simulink model "model1"  (R2024a)
settings: Solver=VariableStepAuto  StartTime=0.0  StopTime=simulation_time  RelTol=1e-3
values from neighbouring files (symbols this model uses):
  dq_0 = zeros(n, 1)    [example.m]
  path = @(t) circle_center + u_circle_plane*radius*cos((t/T) * (2*pi)) + v_circle_plane*radius*sin((t/T) * (2*pi))    [example.m]
  path_ddot = @(t) -u_circle_plane*radius*(2*pi/T)*(2*pi/T)*cos((t/T) * (2*pi)) - v_circle_plane*radius*(2*pi/T)*(2*pi/T)*sin((t/T) * (2*pi))    [example.m]
  path_dot = @(t) -u_circle_plane*radius*(2*pi/T)*sin((t/T) * (2*pi)) + v_circle_plane*radius*(2*pi/T)*cos((t/T) * (2*pi))    [example.m]
  q_0 = randn(n, 1)    [example.m]
  robot_model = importrobot("../robot_model/kuka-lwr-4plus/model1.urdf", 'DataFormat', 'column')    [example.m]
undefined symbols (not defined in the file or in its folder): torque_low_bound, torque_up_bound, X, Y, Z
libraries: sm_lib x74, nesl_utility x8, robotmaniplib x4
(part 3 of 5)

== matlab function model1/MATLAB Function4 ==
  data: currJointPos input; M_num output
function M_num = M_num1(currJointPos)
%M_num1
%    M_num = M_num1(Q2,Q3,Q4,Q5,Q6,Q7)

%    This function was generated by the Symbolic Math Toolbox version 24.1.
%    01-Jul-2024 12:17:03

q2 = currJointPos(2);
q3 = currJointPos(3);
q4 = currJointPos(4);
q5 = currJointPos(5);
q6 = currJointPos(6);
q7 = currJointPos(7);

t2 = cos(q2);
t3 = cos(q3);
t4 = cos(q4);
t5 = cos(q5);
t6 = cos(q6);
t7 = cos(q7);
t8 = sin(q2);
t9 = sin(q3);
t10 = sin(q4);
t11 = sin(q5);
t12 = sin(q6);
t13 = sin(q7);
t14 = t3.^2;
t15 = t4.^2;
t16 = t5.^2;
t17 = t6.^2;
t18 = t7.^2;
t19 = t8.^2;
t20 = t9.^2;
t21 = t10.^2;
t22 = t11.^2;
t23 = t12.^2;
t24 = t13.^2;
t25 = t2.*t4;
t26 = t3.*t5;
t27 = t4.*t6;
t28 = t5.*t7;
t29 = t2.*t10;
t30 = t3.*t11;
t31 = t4.*t12;
t32 = t5.*t13;
t33 = t9.*(2.0./5.0);
t34 = t8.*t9.*t11;
t35 = t9.*t10.*t12;
t36 = t10.*t11.*t13;
t37 = t3.*t4.*t8;
t38 = t4.*t5.*t9;
t39 = t5.*t6.*t10;
t40 = t6.*t7.*t11;
t41 = t3.*t8.*t10;
t42 = t5.*t8.*t9;
t43 = t4.*t9.*t11;
t44 = t6.*t9.*t10;
t45 = t5.*t10.*t12;
t46 = t7.*t10.*t11;
t47 = t6.*t11.*t13;
t48 = t3.*t4.*(2.0./5.0);
t49 = t3.*t8.*(2.0./5.0);
t50 = t3.*t10.*(2.0./5.0);
t53 = t3.*(7.0./1.0e+2);
t57 = t4.*t9.*(3.0./5.0e+1);
t58 = t9.*t11.*(-2.0./5.0);
t59 = t9.*t10.*(3.0./5.0e+1);
t60 = t2.*(1.3e+1./1.0e+2);
t61 = t4.*(3.1e+1./2.5e+2);
t69 = t3.*t4.*(7.0./1.25e+2);
t72 = t4.*t9.*(7.0./1.0e+2);
t74 = t8.*t9.*(2.3e+1./5.0e+1);
t75 = t8.*t9.*(7.0./1.0e+2);
t76 = t2.*1.68e-2;
t77 = t4.*1.68e-2;
t78 = t3.*4.2e-3;
t79 = t2.*7.8e-3;
t80 = t6.*1.2e-4;
t92 = t8.*t9.*t10.*(-2.0./5.0);
t95 = t7.*t11.*(3.9e+1./1.0e+2);
t97 = t10.*t11.*(3.9e+1./1.0e+2);
t98 = t11.*t13.*(3.9e+1./1.0e+2);
t99 = t9.*t10.*(3.1e+1./2.5e+2);
t102 = t3.*1.352e-1;
t104 = t3.*t6.*t10.*(-2.0./5.0);
t114 = t9.*t11.*(6.2e+1./6.25e+2);
t115 = t9.*t10.*1.68e-2;
t116 = t8.*t9.*4.2e-3;
t117 = t9.*t10.*4.2e-3;
t118 = t11.*t12.*1.2e-4;
t125 = t4.*t8.*t9.*(7.0./1.25e+2);
t130 = t8.*t9.*1.352e-1;
t132 = t8.*t9.*5.1e-3;
t133 = t9.*t10.*5.1e-3;
t135 = t5.*9.672e-2;
t173 = t10.*t11.*9.672e-2;
t261 = t3.*1.083333333335e-2;
t267 = t8.*t9.*1.083333333335e-2;
t289 = t5.*2.6708333333367e-3;
t291 = t3.*3.14666666667e-2;
t303 = t2.*7.94666666667e-2;
t308 = t10.*t11.*2.6708333333367e-3;
t309 = t8.*t9.*3.14666666667e-2;
t329 = t3.*t8.*t9.*5.065666666667e-1;
t339 = t4.*t9.*t10.*1.603599999999999e-2;
t352 = t6.*t11.*t12.*5.33333333333e-5;
t358 = t4.*7.50255000000367e-2;
t377 = t9.*t10.*7.50255000000367e-2;
t402 = t5.*t10.*t11.*7.12080000000333e-2;
t51 = t5.*t33;
t52 = t11.*t33;
t54 = t25.*(3.0./5.0e+1);
t55 = -t50;
t56 = t29.*(3.0./5.0e+1);
t62 = -t37;
t63 = -t39;
t65 = -t43;
t68 = -t47;
t70 = t8.*t10.*t33;
t71 = t29.*(7.0./1.0e+2);
t73 = -t59;
t81 = t4.*t26.*(2.0./5.0);
t82 = t8.*t26.*(2.0./5.0);
t83 = t4.*t30.*(2.0./5.0);
t85 = t4.*t8.*t33;
t86 = t8.*t30.*(2.0./5.0);
t87 = t12.*t50;
t88 = -t69;
t89 = t26.*(3.9e+1./1.0e+2);
t90 = t25.*(3.1e+1./2.5e+2);
t91 = t26.*1.5e-3;
t94 = t30.*(3.9e+1./1.0e+2);
t96 = t30.*(3.1e+1./2.5e+2);
t100 = -t76;
t101 = -t77;
t105 = t37.*(3.0./5.0e+1);
t107 = t41.*(3.0./5.0e+1);
t108 = t25.*1.68e-2;
t109 = t25.*4.2e-3;
t110 = t4.*t78;
t111 = t3.*t79;
t112 = t27.*1.2e-4;
t113 = t27.*6.0e-5;
t123 = t37.*(7.0./1.0e+2);
t127 = t25.*5.1e-3;
t128 = t34.*(3.9e+1./1.0e+2);
t129 = t34.*(3.1e+1./2.5e+2);
t131 = -t117;
t134 = -t118;
t136 = t25+t41;
t137 = t30+t38;
t138 = t27+t45;
t139 = t32+t40;
t140 = t8.*t38.*(-2.0./5.0);
t141 = t6.*t28.*(3.9e+1./1.0e+2);
t142 = t8.*t44.*(-2.0./5.0);
t143 = t38.*(3.9e+1./1.0e+2);
t144 = t10.*t28.*(3.9e+1./1.0e+2);
t145 = t6.*t32.*(3.9e+1./1.0e+2);
t146 = t38.*(3.1e+1./2.5e+2);
t147 = -t125;
t148 = t42.*(3.9e+1./1.0e+2);
t149 = t43.*(3.9e+1./1.0e+2);
t150 = t10.*t32.*(3.9e+1./1.0e+2);
t151 = t41.*(3.1e+1./2.5e+2);
t152 = t42.*1.5e-3;
t153 = t43.*1.5e-3;
t154 = -t133;
t156 = t4.*t26.*(6.2e+1./6.25e+2);
t157 = t25.*t80;
t160 = t8.*t30.*(6.2e+1./6.25e+2);
t161 = t41.*1.68e-2;
t164 = t41.*4.2e-3;
t165 = t4.*t116;
t166 = t44.*1.2e-4;
t167 = t12.*t30.*1.2e-4;
t168 = t45.*1.2e-4;
t169 = t44.*6.0e-5;
t170 = t45.*6.0e-5;
t171 = t26.*9.672e-2;
t172 = t4.*t135;
t178 = t10.*t40.*(3.9e+1./1.0e+2);
t180 = t6.*t36.*(3.9e+1./1.0e+2);
t183 = t41.*5.1e-3;
t191 = t8.*t38.*(6.2e+1./6.25e+2);
t192 = t41.*t80;
t193 = t5.*t12.*t29.*1.2e-4;
t194 = t5.*t9.*t31.*1.2e-4;
t196 = t12.*t34.*1.2e-4;
t197 = t33+t72;
t199 = t42.*9.672e-2;
t200 = t11.*t29.*9.672e-2;
t201 = t43.*9.672e-2;
t202 = t50+t57;
t206 = t8.*t26.*t31.*1.2e-4;
t213 = t4.*t8.*t30.*9.672e-2;
t215 = t60+t74;
t217 = t61+t97;
t225 = t79+t132;
t268 = t29.*1.533333333335e-2;
t270 = t30.*2.170133333335e-2;
t271 = t25.*2.080133333335e-2;
t272 = t26.*1.302083333335e-3;
t273 = t27.*1.302083333335e-3;
t274 = t31.*1.302083333335e-3;
t278 = t37.*1.533333333335e-2;
t279 = t38.*2.170133333335e-2;
t280 = t34.*2.170133333335e-2;
t281 = t41.*2.080133333335e-2;
t282 = t39.*1.302083333335e-3;
t283 = t42.*1.302083333335e-3;
t284 = t43.*1.302083333335e-3;
t285 = t44.*1.302083333335e-3;
t286 = t45.*1.302083333335e-3;
t287 = t35.*1.302083333335e-3;
t292 = t28.*3.333333333335e-5;
t293 = t32.*3.333333333335e-5;
t301 = -t289;
t302 = -t291;
t306 = t26.*2.6708333333367e-3;
t310 = t40.*3.333333333335e-5;
t312 = t46.*3.333333333335e-5;
t313 = t47.*3.333333333335e-5;
t314 = t36.*3.333333333335e-5;
t319 = -t308;
t320 = -t309;
t326 = t42.*2.6708333333367e-3;
t327 = t11.*t29.*2.6708333333367e-3;
t328 = t43.*2.6708333333367e-3;
t335 = -t329;
t342 = t4.*t8.*t30.*2.6708333333367e-3;
t343 = -t339;
t348 = t4.*t17.*5.33333333333e-5;
t364 = -t352;
t368 = t9.*t10.*t17.*5.33333333333e-5;
t370 = t6.*t12.*t30.*5.33333333333e-5;
t371 = t11.*t12.*t27.*5.33333333333e-5;
t372 = t12.*t39.*5.33333333333e-5;
t375 = t17.*t25.*5.33333333333e-5;
t384 = t25.*7.50255000000367e-2;
t385 = -t377;
t390 = t5.*t6.*t12.*t29.*5.33333333333e-5;
t391 = t5.*t9.*t12.*t27.*5.33333333333e-5;
t392 = t6.*t12.*t34.*5.33333333333e-5;
t394 = t17.*t41.*5.33333333333e-5;
t395 = t5.*t10.*t11.*t17.*5.33333333333e-5;
t401 = t41.*7.50255000000367e-2;
t403 = t8.*t12.*t26.*t27.*5.33333333333e-5;
t405 = -t402;
t93 = -t71;
t103 = -t82;
t106 = -t86;
t119 = t4.*t8.*t51;
t120 = t4.*t8.*t52;
t122 = -t105;
t124 = t12.*t70;
t126 = -t108;
t155 = -t141;
t158 = -t148;
t159 = -t149;
t163 = -t153;
t174 = t29+t62;
t175 = t26+t65;
t176 = t31+t63;
t177 = t28+t68;
t179 = -t156;
t181 = -t160;
t182 = -t161;
t184 = -t166;
t186 = -t171;
t187 = t6.*t136;
t188 = t6.*t137;
t189 = t12.*t136;
t190 = t12.*t137;
t195 = -t180;
t198 = -t191;
t211 = -t199;
t212 = -t206;
t216 = -t213;
t226 = t10.*t197.*(7.0./5.0e+1);
t227 = t95+t145;
t229 = t78+t154;
t230 = t10.*t202.*(3.0./2.5e+1);
t238 = t112+t168;
t239 = t113+t170;
t240 = t48+t53+t73;
t241 = t3.*t225;
t244 = t3.*t215.*(2.3e+1./2.5e+1);
t246 = t150+t178;
t258 = t55+t96+t146;
t275 = t54+t75+t85+t107;
t276 = t116+t127+t183;
t288 = t51+t83+t94+t143;
t290 = -t278;
t297 = -t282;
t298 = -t283;
t299 = -t284;
t300 = -t285;
t321 = -t312;
t322 = -t313;
t332 = -t327;
t333 = -t328;
t345 = t11.*t137.*2.170133333335e-2;
t353 = t131+t261;
t360 = t5.*t10.*t137.*2.170133333335e-2;
t363 = t9.*t10.*t136.*2.080133333335e-2;
t378 = -t368;
t380 = -t371;
t398 = t4.*t136.*2.590133333335e-2;
t406 = -t403;
t436 = t135+t364;
t438 = t109+t164+t267;
t468 = t270+t279;
t470 = t271+t281;
t472 = t273+t286;
t491 = t293+t310;
t594 = t173+t348+t358+t372;
t203 = t5.*t174;
t204 = t7.*t175;
t205 = t7.*t176;
t207 = t11.*t174;
t209 = t13.*t175;
t210 = t13.*t176;
t218 = t187.*6.0e-5;
t219 = t190.*6.0e-5;
t220 = t35+t188;
t234 = t98+t155;
t235 = t91+t163;
t245 = t4.*t229;
t250 = t144+t195;
t255 = t56+t70+t122;
t256 = t49+t93+t123;
t259 = t4.*t240.*(3.0./2.5e+1);
t264 = t136.*t229;
t294 = t11.*t258.*(3.1e+1./1.25e+2);
t305 = t4.*t276;
t307 = t58+t81+t89+t159;
t311 = t5.*t10.*t258.*(3.1e+1./1.25e+2);
t315 = t167+t184+t194;
t323 = t7.*t288;
t324 = t13.*t288;
t325 = t9.*t10.*t276;
t340 = t4.*t275.*(3.0./2.5e+1);
t350 = -t345;
t354 = t187.*1.302083333335e-3;
t355 = t188.*1.302083333335e-3;
t356 = t189.*1.302083333335e-3;
t357 = t190.*1.302083333335e-3;
t359 = t10.*t174.*1.533333333335e-2;
t365 = t11.*t288.*(1.17e+2./1.0e+2);
t369 = -t363;
t374 = -t239.*(t44-t190);
t379 = t4.*t9.*t174.*1.533333333335e-2;
t381 = t5.*t10.*t288.*(1.17e+2./1.0e+2);
t396 = t8.*t9.*t353;
t407 = t5.*t175.*2.802083333335e-3;
t414 = t10.*t11.*t175.*2.802083333335e-3;
t442 = t240.*t275.*2.0;
t443 = t3.*t438;
t459 = t11.*t12.*(t44-t190).*1.362083333335e-3;
t466 = t157+t192+t193+t196+t212;
t471 = t268+t290;
t475 = t272+t299;
t476 = t274+t297;
t477 = t11.*t468;
t478 = t4.*t470;
t483 = t5.*t10.*t468;
t486 = t9.*t10.*t470;
t498 = t292+t322;
t507 = t306+t333;
t534 = -t472.*(t44-t190);
t571 = t326+t332+t342;
t606 = t101+t172+t380+t395+t405;
t616 = t114+t179+t186+t201+t370+t378+t385+t391;
t617 = t181+t198+t200+t211+t216+t375+t384+t390+t392+t394+t401+t406;
t221 = t203.*(3.9e+1./1.0e+2);
t222 = t203.*(3.1e+1./2.5e+2);
t223 = t207.*(3.9e+1./1.0e+2);
t224 = t207.*1.5e-3;
t231 = t34+t203;
t233 = t36+t205;
t236 = t7.*t220;
t237 = t13.*t220;
t249 = t5.*t235;
t253 = t10.*t11.*t235;
t265 = t10.*t255.*(3.0./2.5e+1);
t266 = t10.*t256.*(7.0./5.0e+1);
t304 = -t294;
t316 = t11.*t12.*(t169-t219);
t334 = t6.*t307;
t336 = t12.*t307;
t338 = -t325;
t347 = t197.*t256.*2.0;
t349 = t202.*t255.*2.0;
t361 = t203.*2.170133333335e-2;
t366 = -t138.*(t169-t219);
t367 = -t356;
t373 = -t365;
t376 = t207.*1.302083333335e-3;
t386 = t204.*3.333333333335e-5;
t387 = t205.*3.333333333335e-5;
t388 = t209.*3.333333333335e-5;
t389 = t210.*3.333333333335e-5;
t393 = t99+t307;
t399 = t235.*(t42-t207);
t412 = -t407;
t418 = -t414;
t428 = t6.*t11.*t220.*1.302083333335e-3;
t440 = t13.*(t42-t207).*(-3.333333333335e-5);
t448 = t5.*(t42-t207).*(-2.802083333335e-3);
t456 = t10.*t11.*(t42-t207).*(-2.802083333335e-3);
t481 = t10.*t471;
t484 = -t477;
t489 = t5.*t475;
t492 = t4.*t9.*t471;
t496 = -t486;
t500 = t10.*t11.*t475;
t512 = t287+t355;
t513 = t300+t357;
t532 = t220.*t476;
t540 = t475.*(t42-t207);
t228 = -t223;
t247 = t6.*t231;
t248 = t12.*t231;
t254 = -t249;
t257 = -t253;
t269 = -t266;
t277 = -t5.*(t152-t224);
t295 = -t10.*t11.*(t152-t224);
t318 = t209+t236;
t341 = t92+t129+t222;
t351 = -t347;
t397 = -t386;
t400 = t175.*(t152-t224);
t409 = t87+t334;
t413 = t104+t336;
t415 = t103+t120+t128+t221;
t424 = t11.*t231.*2.170133333335e-2;
t425 = t5.*t393.*(3.9e+1./5.0e+1);
t432 = t236.*3.333333333335e-5;
t433 = t237.*3.333333333335e-5;
t434 = -t428;
t435 = t5.*t10.*t231.*2.170133333335e-2;
t462 = t217.*t393.*2.0;
t482 = t90+t106+t140+t151+t158+t223;
t501 = -t489;
t505 = -t500;
t511 = t280+t361;
t514 = t298+t376;
t517 = t6.*t11.*t512;
t519 = t314+t387;
t520 = t11.*t12.*t513;
t522 = t321+t389;
t528 = t231.*t468;
t533 = t138.*t513;
t535 = t176.*t512;
t536 = -t532;
t562 = -t498.*(t204-t237);
t260 = t248.*6.0e-5;
t317 = t187+t248;
t344 = -t7.*(t189-t247);
t362 = t7.*(t189-t247);
t404 = t11.*t341.*(3.1e+1./1.25e+2);
t410 = t5.*t10.*t341.*(3.1e+1./1.25e+2);
t416 = t86+t119+t148+t228;
t417 = t7.*t409;
t419 = t13.*t409;
t421 = t7.*t415;
t423 = t13.*t415;
t426 = -t424;
t429 = t247.*1.302083333335e-3;
t430 = t248.*1.302083333335e-3;
t431 = -t425;
t441 = t5.*t6.*t409.*(3.9e+1./1.0e+2);
t445 = t11.*t415.*(1.17e+2./1.0e+2);
t446 = t5.*t12.*t413.*(1.17e+2./2.5e+2);
t451 = t5.*t10.*t415.*(1.17e+2./1.0e+2);
t452 = t6.*t10.*t11.*t409.*(-3.9e+1./1.0e+2);
t455 = t10.*t11.*t12.*t413.*(1.17e+2./2.5e+2);
t465 = -t462;
t474 = t258.*t341.*2.0;
t499 = t6.*t11.*(t189-t247).*1.302083333335e-3;
t508 = t5.*t482.*(3.9e+1./5.0e+1);
t515 = t11.*t511;
t516 = t5.*t10.*t511;
t521 = t5.*t514;
t523 = -t517;
t524 = t10.*t11.*t514;
t525 = -t520;
t526 = t288.*t415.*3.0;
t529 = t137.*t511;
t530 = t217.*t482.*2.0;
t537 = -t535;
t539 = t175.*t514;
t544 = t388+t432;
t546 = t397+t433;
t554 = t318.*t491;
t556 = t476.*(t189-t247);
t573 = -t512.*(t189-t247);
t575 = t393.*t482.*2.0;
t580 = t318.*t519;
t586 = t522.*(t204-t237);
t589 = -t498.*(t7.*(t42-t207)+t13.*(t189-t247));
t593 = -t177.*(t7.*(t42-t207).*3.333333333335e-5+t13.*(t189-t247).*3.333333333335e-5);
t602 = (t7.*(t42-t207).*3.333333333335e-5+t13.*(t189-t247).*3.333333333335e-5).*(t46-t210);
t604 = t522.*(t7.*(t42-t207)+t13.*(t189-t247));
t610 = (t7.*(t42-t207).*3.333333333335e-5+t13.*(t189-t247).*3.333333333335e-5).*(t204-t237);
t408 = -t404;
t411 = t218+t260;
t420 = t6.*t416;
t422 = t12.*t416;
t444 = -t441;
t447 = -t445;
t450 = -t446;
M_num = ft_1({t10,t100,t102,t11,t110,t111,t115,t12,t124,t126,t13,t130,t134,t136,t137,t138,t139,t14,t142,t147,t15,t152,t16,t165,t169,t17,t174,t175,t176,t177,t18,t182,t189,t19,t190,t197,t2,t20,t202,t204,t207,t21,t210,t215,t217,t219,t22,t220,t224,t225,t226,t227,t229,t23,t230,t231,t233,t234,t235,t237,t238,t239,t24,t240,t241,t244,t245,t246,t247,t250,t254,t255,t256,t257,t258,t259,t264,t265,t269,t275,t276,t277,t288,t295,t3,t301,t302,t303,t304,t305,t311,t315,t316,t317,t318,t319,t320,t323,t324,t335,t338,t340,t341,t343,t344,t349,t350,t351,t353,t354,t359,t360,t362,t366,t367,t369,t373,t374,t379,t381,t393,t396,t398,t399,t400,t408,t409,t410,t411,t412,t413,t415,t417,t418,t419,t42,t420,t421,t422,t423,t426,t429,t430,t431,t434,t435,t436,t438,t44,t440,t442,t443,t444,t447,t448,t450,t451,t452,t455,t456,t459,t46,t465,t466,t468,t470,t471,t472,t474,t475,t476,t478,t481,t482,t483,t484,t491,t492,t496,t498,t499,t5,t501,t505,t507,t508,t511,t512,t513,t514,t515,t516,t519,t521,t522,t523,t524,t525,t526,t528,t529,t530,t533,t534,t536,t537,t539,t540,t544,t546,t554,t556,t562,t571,t573,t575,t580,t586,t589,t593,t594,t6,t602,t604,t606,t610,t616,t617,t7,t8,t80,t88,t9});
end
function M_num = ft_1(ct)
[t10,t100,t102,t11,t110,t111,t115,t12,t124,t126,t13,t130,t134,t136,t137,t138,t139,t14,t142,t147,t15,t152,t16,t165,t169,t17,t174,t175,t176,t177,t18,t182,t189,t19,t190,t197,t2,t20,t202,t204,t207,t21,t210,t215,t217,t219,t22,t220,t224,t225,t226,t227,t229,t23,t230,t231,t233,t234,t235,t237,t238,t239,t24,t240,t241,t244,t245,t246,t247,t250,t254,t255,t256,t257,t258,t259,t264,t265,t269,t275,t276,t277,t288,t295,t3,t301,t302,t303,t304,t305,t311,t315,t316,t317,t318,t319,t320,t323,t324,t335,t338,t340,t341,t343,t344,t349,t350,t351,t353,t354,t359,t360,t362,t366,t367,t369,t373,t374,t379,t381,t393,t396,t398,t399,t400,t408,t409,t410,t411,t412,t413,t415,t417,t418,t419,t42,t420,t421,t422,t423,t426,t429,t430,t431,t434,t435,t436,t438,t44,t440,t442,t443,t444,t447,t448,t450,t451,t452,t455,t456,t459,t46,t465,t466,t468,t470,t471,t472,t474,t475,t476,t478,t481,t482,t483,t484,t491,t492,t496,t498,t499,t5,t501,t505,t507,t508,t511,t512,t513,t514,t515,t516,t519,t521,t522,t523,t524,t525,t526,t528,t529,t530,t533,t534,t536,t537,t539,t540,t544,t546,t554,t556,t562,t571,t573,t575,t580,t586,t589,t593,t594,t6,t602,t604,t606,t610,t616,t617,t7,t8,t80,t88,t9] = ct{:};
t453 = t239.*t317;
t457 = -t455;
t479 = -t317.*(t169-t219);
t494 = t362.*3.333333333335e-5;
t509 = t11.*t12.*t317.*1.362083333335e-3;
t518 = -t515;
t527 = t323+t419;
t541 = -t539;
t542 = t354+t430;
t543 = t367+t429;
t550 = t317.*t472;
t555 = t139.*t544;
t559 = -t554;
t563 = t177.*t546;
t565 = t234.*(t324-t417).*(-1.0./5.0);
t569 = t317.*t513;
t574 = (t246.*(t324-t417))./5.0;
t577 = -t575;
t579 = t233.*t544;
t582 = -t580;
t585 = t546.*(t46-t210);
t592 = -t491.*(t344+t13.*(t42-t207));
t603 = -t519.*(t344+t13.*(t42-t207));
t605 = -t602;
t607 = -t546.*(t7.*(t42-t207)+t13.*(t189-t247));
t612 = t544.*(t344+t13.*(t42-t207));
t427 = t11.*t12.*t411;
t454 = t138.*t411;
t460 = t124+t420;
t461 = t142+t422;
t480 = -t411.*(t44-t190);
t510 = -t509;
t545 = t11.*t12.*t542;
t547 = t6.*t11.*t543;
t551 = t138.*t542;
t553 = t176.*t543;
t560 = -t555;
t561 = (t227.*t527)./5.0;
t567 = (t250.*t527)./5.0;
t568 = t220.*t543;
t572 = -t542.*(t44-t190);
t581 = -t579;
t588 = t440+t494;
t437 = -t427;
t463 = t7.*t460;
t464 = t13.*t460;
t485 = t5.*t6.*t460.*(3.9e+1./1.0e+2);
t497 = t5.*t12.*t461.*(1.17e+2./2.5e+2);
t502 = t6.*t10.*t11.*t460.*(-3.9e+1./1.0e+2);
t504 = t10.*t11.*t12.*t461.*(1.17e+2./2.5e+2);
t548 = -t545;
t549 = -t547;
t557 = -t553;
t558 = t409.*t460;
t564 = -t561;
t566 = t413.*t461.*(6.0./5.0);
t590 = t139.*t588;
t600 = t233.*t588;
t608 = t318.*t588;
t619 = t102+t110+t226+t230+t245+t257+t259+t311+t343+t360+t366+t374+t381+t418+t452+t457+t465+t483+t505+t533+t534+t536+t537+t567+t574+t581+t582+t585+t586;
t467 = -t463;
t490 = -t485;
t503 = -t497;
t506 = -t504;
t576 = t421+t464;
t611 = -t608;
t618 = t88+t115+t254+t302+t304+t316+t350+t373+t412+t431+t434+t444+t450+t459+t484+t501+t523+t525+t559+t560+t562+t563+t564+t565;
t578 = t423+t467;
t591 = (t227.*t576)./5.0;
t598 = (t250.*t576)./5.0;
t613 = (t527.*t576)./5.0;
t595 = -t591;
t596 = (t234.*t578)./5.0;
t599 = (t246.*t578)./5.0;
t615 = (t578.*(t324-t417))./5.0;
t597 = -t596;
t621 = t130+t165+t265+t269+t295+t303+t305+t340+t359+t398+t410+t435+t451+t453+t454+t456+t478+t481+t502+t506+t516+t524+t530+t550+t551+t556+t557+t598+t599+t600+t603+t604+t605;
t622 = t100+t111+t241+t244+t264+t335+t338+t349+t351+t369+t379+t396+t399+t400+t442+t443+t474+t479+t480+t492+t496+t526+t528+t529+t540+t541+t558+t566+t568+t569+t572+t573+t577+t607+t610+t611+t612+t613+t615;
t620 = t126+t147+t182+t277+t320+t408+t426+t437+t447+t448+t490+t499+t503+t508+t510+t518+t521+t548+t549+t589+t590+t592+t593+t595+t597;
et1 = t19.*4.76666666667e-2-t588.*(t344+t13.*(t42-t207)).*2.0+(t7.*(t42-t207)+t13.*(t189-t247)).*(t7.*(t42-t207).*3.333333333335e-5+t13.*(t189-t247).*3.333333333335e-5).*2.0;
et2 = t14.*t19.*5.116666666667e-1+t136.*t276.*2.0+t136.*t470.*2.0+t174.*t471.*2.0+t317.*t411.*2.0+t231.*t511.*2.0+t317.*t542.*2.0+t2.*(t2.*2.283333333335e-2+t8.*t9.*7.8e-3).*2.0-t514.*(t42-t207).*2.0-t543.*(t189-t247).*2.0+(t42-t207).*(t152-t224).*2.0+t2.^2.*1.74e-2+t215.^2.*2.0+t255.^2.*2.0+t256.^2.*2.0+t275.^2.*2.0+t341.^2.*2.0+t415.^2.*3.0+t460.^2;
et3 = t461.^2.*(6.0./5.0)+t482.^2.*2.0+t576.^2./5.0+t578.^2./5.0+t8.*t9.*t225.*2.0+t8.*t9.*t438.*2.0+7.94666666667e-2;
et4 = t14.*4.334e-1+t20.*5.116666666667e-1+(t324-t417).^2./5.0+t15.*t20.*3.06666666667e-2+t20.*t21.*4.16026666667e-2+t3.*t353.*2.0+t175.*t235.*2.0+t137.*t468.*2.0+t175.*t475.*2.0+t220.*t512.*2.0+t318.*t544.*2.0-t513.*(t44-t190).*2.0-t546.*(t204-t237).*2.0+(t44-t190).*(t169-t219).*2.0;
et5 = t197.^2.*2.0+t202.^2.*2.0+t240.^2.*2.0+t258.^2.*2.0+t288.^2.*3.0+t393.^2.*2.0+t409.^2+t413.^2.*(6.0./5.0)+t527.^2./5.0-t9.*t10.*t229.*2.0+3.14666666667e-2;
et6 = t15.*5.90026666667e-2+t21.*4.76666666667e-2+t16.*t21.*5.304546666667e-1+t21.*t22.*5.60416666667e-3+t138.*t239.*2.0+t138.*t472.*2.0+t176.*t476.*2.0+t233.*t519.*2.0;
et7 = t522.*(t46-t210).*-2.0+t217.^2.*2.0+t246.^2./5.0+t250.^2./5.0+t17.*t21.*t22.*1.521e-1+t21.*t22.*t23.*1.8252e-1+7.94666666667e-2;
et8 = t16.*3.0980416666667e-1+t22.*5.304546666667e-1+t16.*t17.*1.521e-1+t16.*t23.*1.8252e-1+t17.*t22.*2.60416666667e-3;
et9 = t22.*t23.*2.72416666667e-3+t139.*t491.*2.0+t177.*t498.*2.0+t227.^2./5.0+t234.^2./5.0+3.14666666667e-2;
et10 = t17.*2.72416666667e-3+t23.*2.60416666667e-3+t18.*t23.*6.66666666667e-5+t23.*t24.*6.66666666667e-5;
et11 = 7.23546666667e-2;
M_num = reshape([et1+et2+et3,t622,t621,t620,t617,t571,t466,t622,et4+et5,t619,t618,t616,t507,t315,t621,t619,et6+et7,t606,t594,t319,t238,t620,t618,t606,et8+et9,t436,t301,t134,t617,t616,t594,t436,et10+et11,0.0,t80,t571,t507,t319,t301,0.0,t18.*6.66666666667e-5+t24.*6.66666666667e-5+2.60416666667e-3,0.0,t466,t315,t238,t134,t80,0.0,1.2e-4],[7,7]);
end
